simulink model "stm32_step3_DDS_10kHz_a"  (R2018a)
settings: Solver=FixedStepDiscrete  StartTime=0.0  StopTime=inf  RelTol=1e-3
PreLoadFcn:
  | waijung.modelPreload; % Required for working with Waijung Blockset. Do not remove.
undefined symbols (not defined in the file or in its folder): HSEOSC, Link, LQFP176, ST, STM32F417IG
libraries: simulink x4, stm32f4_io_lib x4, stm32f4_device_config_lib x1, stm32f4_tim_lib x1
(part 2 of 2)

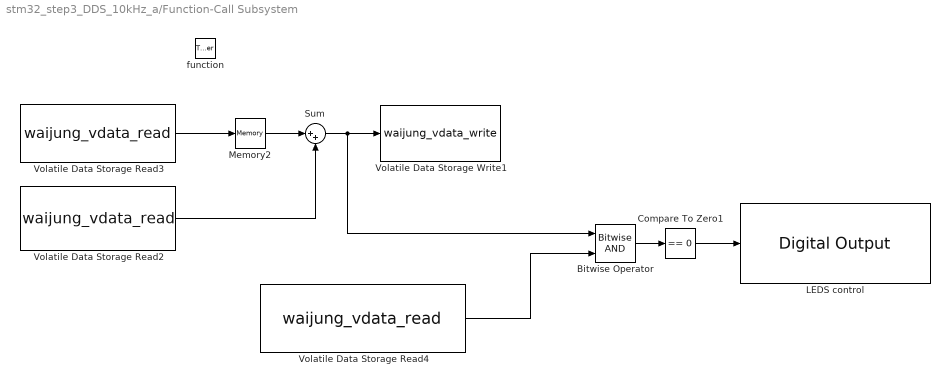
== system stm32_step3_DDS_10kHz_a/Function-Call Subsystem ==
  function : TriggerPort  TriggerType=function-call  VariantControl=Variant
  Bitwise Operator : simulink/Logic and Bit Operations/Bitwise Operator  logicop=AND  UseBitMask=off  NumInputPorts=2  BitMask=bin2dec('11011001')  BitMaskRealWorld=Stored Integer
  Compare To Zero1 : simulink/Logic and Bit Operations/Compare To Zero  relop===  OutDataTypeStr=boolean
  LEDS control : stm32f4_io_lib/Digital Output  use_bitband=on  port=D  speed=100  porttype=Push Pull  porttypestr=PP  use_pin0=off  use_pin1=off  use_pin2=off  use_pin3=off  use_pin4=off  use_pin5=off  use_pin6=off  use_pin7=off  use_pin8=off  use_pin9=off  use_pin10=off  use_pin11=off  use_pin12=off  use_pin13=off  use_pin14=off  use_pin15=on  pinstr=GPIO_Pin_15  usedpinarray="[0  0  0  0  0  0  0  0  0  0  0  0  0  0  0  1]"  bitbandingstr="#define FunctionCallSubsystemLEDScontrol_D15 Peripheral_BB(GPIOD->ODR, 15)  /* Output pin */"  sampletime=-1  sampletimestr=-1  blockid=FunctionCallSubsystemLEDScontrol  enablecustomportlabel=off  globalinit=off  cinputportlabel=In1, In2  coutputportlabel=0
      settings: SourceProductName=Waijung Blockset
  Memory2 : Memory  InheritSampleTime=on
  Sum : Sum  Inputs=|++
  Volatile Data Storage Read2 : S-Function  FunctionName=waijung_vdata_read  Parameters=storagename,varname,sampletime,sampletimestr,blockid,storagetype,storagetypestr  SFunctionDeploymentMode=off  EnableBusSupport=off  mask(waijung_vdata_read){storagename=DDS_TUNE, varname=VolatileDataStorage3_DDS_TUNE, sampletime=-1, sampletimestr=-1, blockid=FunctionCallSubsystemVolatileDataStorageRead2, storagetype=uint16, storagetypestr=uint16_t}
      mask prompts: storagename "Storage Name"; varname "Variable name"; sampletime "Sample time (sec)"; sampletimestr "Compiled sample time (sec) in string"; storagetype "Data type"; storagetypestr "Data type string"
      mask help: This block implements read data from a buffer.
      mask init:
      | waijung_vdata_read_callback('init');
      mask Help: web(fullfile(waijungdocroot,'Volatile_Data_Storage_Read.htm'))
      mask TypeOptions storagename: LEDfreq | DDS_ACC | DDS_MASK | DDS_TUNE | SPEED
      mask Callback storagename: waijung_vdata_read_callback('storagename');
      mask Callback varname: waijung_vdata_read_callback('varname');
      mask Callback sampletime: waijung_vdata_read_callback('sampletime');
      mask Callback sampletimestr: waijung_vdata_read_callback('sampletimestr');
      mask Callback blockid: waijung_vdata_read_callback('blockid');
      mask Callback storagetype: waijung_vdata_read_callback('storagetype');
      mask Display: text(0.05, 0.5, 'Buffer: DDS_TUNE','ver','middle','hor','left');port_label('output',1,'D1(uint16)')
  Volatile Data Storage Read3 : S-Function  FunctionName=waijung_vdata_read  Parameters=storagename,varname,sampletime,sampletimestr,blockid,storagetype,storagetypestr  SFunctionDeploymentMode=off  EnableBusSupport=off  mask(waijung_vdata_read){storagename=DDS_ACC, varname=VolatileDataStorage1_DDS_ACC, sampletime=-1, sampletimestr=-1, blockid=FunctionCallSubsystemVolatileDataStorageRead3, storagetype=uint16, storagetypestr=uint16_t}
      mask prompts: storagename "Storage Name"; varname "Variable name"; sampletime "Sample time (sec)"; sampletimestr "Compiled sample time (sec) in string"; storagetype "Data type"; storagetypestr "Data type string"
      mask help: This block implements read data from a buffer.
      mask init:
      | waijung_vdata_read_callback('init');
      mask Help: web(fullfile(waijungdocroot,'Volatile_Data_Storage_Read.htm'))
      mask TypeOptions storagename: LEDfreq | DDS_ACC | DDS_MASK | DDS_TUNE | SPEED
      mask Callback storagename: waijung_vdata_read_callback('storagename');
      mask Callback varname: waijung_vdata_read_callback('varname');
      mask Callback sampletime: waijung_vdata_read_callback('sampletime');
      mask Callback sampletimestr: waijung_vdata_read_callback('sampletimestr');
      mask Callback blockid: waijung_vdata_read_callback('blockid');
      mask Callback storagetype: waijung_vdata_read_callback('storagetype');
      mask Display: text(0.05, 0.5, 'Buffer: DDS_ACC','ver','middle','hor','left');port_label('output',1,'D1(uint16)')
  Volatile Data Storage Read4 : S-Function  FunctionName=waijung_vdata_read  Parameters=storagename,varname,sampletime,sampletimestr,blockid,storagetype,storagetypestr  SFunctionDeploymentMode=off  EnableBusSupport=off  mask(waijung_vdata_read){storagename=DDS_MASK, varname=VolatileDataStorage2_DDS_MASK, sampletime=-1, sampletimestr=-1, blockid=FunctionCallSubsystemVolatileDataStorageRead4, storagetype=uint16, storagetypestr=uint16_t}
      mask prompts: storagename "Storage Name"; varname "Variable name"; sampletime "Sample time (sec)"; sampletimestr "Compiled sample time (sec) in string"; storagetype "Data type"; storagetypestr "Data type string"
      mask help: This block implements read data from a buffer.
      mask init:
      | waijung_vdata_read_callback('init');
      mask Help: web(fullfile(waijungdocroot,'Volatile_Data_Storage_Read.htm'))
      mask TypeOptions storagename: LEDfreq | DDS_ACC | DDS_MASK | DDS_TUNE | SPEED
      mask Callback storagename: waijung_vdata_read_callback('storagename');
      mask Callback varname: waijung_vdata_read_callback('varname');
      mask Callback sampletime: waijung_vdata_read_callback('sampletime');
      mask Callback sampletimestr: waijung_vdata_read_callback('sampletimestr');
      mask Callback blockid: waijung_vdata_read_callback('blockid');
      mask Callback storagetype: waijung_vdata_read_callback('storagetype');
      mask Display: text(0.05, 0.5, 'Buffer: DDS_MASK','ver','middle','hor','left');port_label('output',1,'D1(uint16)')
  Volatile Data Storage Write1 : S-Function  FunctionName=waijung_vdata_write  Parameters=storagename,varname,sampletime,sampletimestr,blockid,storagetype,storagetypestr  SFunctionDeploymentMode=off  EnableBusSupport=off  mask(waijung_vdata_write){storagename=DDS_ACC, varname=VolatileDataStorage1_DDS_ACC, sampletime=-1, sampletimestr=-1, blockid=FunctionCallSubsystemVolatileDataStorageWrite1, storagetype=uint16, storagetypestr=uint16_t}
      mask prompts: storagename "Storage Name"; varname "Variable name"; sampletime "Sample time (sec)"; sampletimestr "Compiled sample time (sec) in string"; storagetype "Data type"; storagetypestr "Data type string"
      mask help: This block implements write data to a buffer.
      mask init:
      | waijung_vdata_write_callback('init');
      mask Help: web(fullfile(waijungdocroot,'Volatile_Data_Storage_Write.htm'))
      mask TypeOptions storagename: LEDfreq | DDS_ACC | DDS_MASK | DDS_TUNE | SPEED
      mask Callback storagename: waijung_vdata_write_callback('storagename');
      mask Callback varname: waijung_vdata_write_callback('varname');
      mask Callback sampletime: waijung_vdata_write_callback('sampletime');
      mask Callback sampletimestr: waijung_vdata_write_callback('sampletimestr');
      mask Callback blockid: waijung_vdata_write_callback('blockid');
      mask Callback storagetype: waijung_vdata_write_callback('storagetype');
      mask Display: text(0.95, 0.5, 'Buffer: DDS_ACC','ver','middle','hor','right');port_label('input',1,'D1(uint16)')
  wires:
  Volatile Data Storage Read3/1 -> Memory2/1
  Memory2/1 -> Sum/1
  Volatile Data Storage Read2/1 -> Sum/2
  Sum/1 -> Bitwise Operator/1, Volatile Data Storage Write1/1
  Volatile Data Storage Read4/1 -> Bitwise Operator/2
  Bitwise Operator/1 -> Compare To Zero1/1
  Compare To Zero1/1 -> LEDS control/1

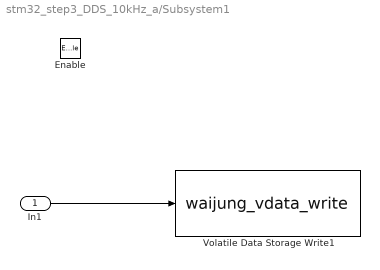
== system stm32_step3_DDS_10kHz_a/Subsystem1 ==
  In1 : Inport
  Enable : EnablePort
  Volatile Data Storage Write1 : S-Function  FunctionName=waijung_vdata_write  Parameters=storagename,varname,sampletime,sampletimestr,blockid,storagetype,storagetypestr  SFunctionDeploymentMode=off  EnableBusSupport=off  mask(waijung_vdata_write){storagename=DDS_MASK, varname=VolatileDataStorage2_DDS_MASK, sampletime=-1, sampletimestr=0.1, blockid=Subsystem1VolatileDataStorageWrite1, storagetype=uint16, storagetypestr=uint16_t}
      mask prompts: storagename "Storage Name"; varname "Variable name"; sampletime "Sample time (sec)"; sampletimestr "Compiled sample time (sec) in string"; storagetype "Data type"; storagetypestr "Data type string"
      mask help: This block implements write data to a buffer.
      mask init:
      | waijung_vdata_write_callback('init');
      mask Help: web(fullfile(waijungdocroot,'Volatile_Data_Storage_Write.htm'))
      mask TypeOptions storagename: LEDfreq | DDS_ACC | DDS_MASK | DDS_TUNE | SPEED
      mask Callback storagename: waijung_vdata_write_callback('storagename');
      mask Callback varname: waijung_vdata_write_callback('varname');
      mask Callback sampletime: waijung_vdata_write_callback('sampletime');
      mask Callback sampletimestr: waijung_vdata_write_callback('sampletimestr');
      mask Callback blockid: waijung_vdata_write_callback('blockid');
      mask Callback storagetype: waijung_vdata_write_callback('storagetype');
      mask Display: text(0.95, 0.5, 'Buffer: DDS_MASK','ver','middle','hor','right');port_label('input',1,'D1(uint16)')
  wires:
  In1/1 -> Volatile Data Storage Write1/1

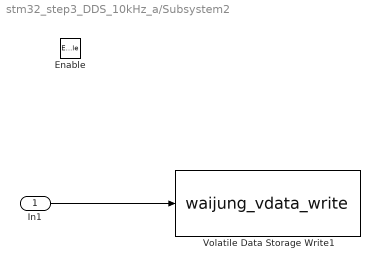
== system stm32_step3_DDS_10kHz_a/Subsystem2 ==
  In1 : Inport
  Enable : EnablePort
  Volatile Data Storage Write1 : S-Function  FunctionName=waijung_vdata_write  Parameters=storagename,varname,sampletime,sampletimestr,blockid,storagetype,storagetypestr  SFunctionDeploymentMode=off  EnableBusSupport=off  mask(waijung_vdata_write){storagename=DDS_TUNE, varname=VolatileDataStorage3_DDS_TUNE, sampletime=-1, sampletimestr=0.1, blockid=Subsystem2VolatileDataStorageWrite1, storagetype=uint16, storagetypestr=uint16_t}
      mask prompts: storagename "Storage Name"; varname "Variable name"; sampletime "Sample time (sec)"; sampletimestr "Compiled sample time (sec) in string"; storagetype "Data type"; storagetypestr "Data type string"
      mask help: This block implements write data to a buffer.
      mask init:
      | waijung_vdata_write_callback('init');
      mask Help: web(fullfile(waijungdocroot,'Volatile_Data_Storage_Write.htm'))
      mask TypeOptions storagename: LEDfreq | DDS_ACC | DDS_MASK | DDS_TUNE | SPEED
      mask Callback storagename: waijung_vdata_write_callback('storagename');
      mask Callback varname: waijung_vdata_write_callback('varname');
      mask Callback sampletime: waijung_vdata_write_callback('sampletime');
      mask Callback sampletimestr: waijung_vdata_write_callback('sampletimestr');
      mask Callback blockid: waijung_vdata_write_callback('blockid');
      mask Callback storagetype: waijung_vdata_write_callback('storagetype');
      mask Display: text(0.95, 0.5, 'Buffer: DDS_TUNE','ver','middle','hor','right');port_label('input',1,'D1(uint16)')
  wires:
  In1/1 -> Volatile Data Storage Write1/1
